simulink model "DiagramaMalhaFechadaForno"  (R2015a)
settings: Solver=ode45  StartTime=0.0  StopTime=15000  RelTol=1e-3
values from neighbouring files (symbols this model uses):
  G = (0.1858/(s + 0.0001438))    [Code50MatLab.m]
libraries: simulink x1
settings Model: Creator=Raian  LastModifiedBy=Emiliano

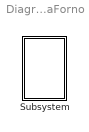
== system DiagramaMalhaFechadaForno ==
  Subsystem : Subsystem

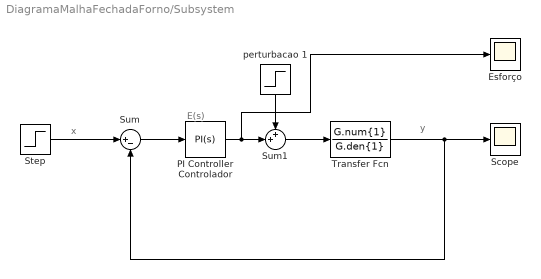
== system DiagramaMalhaFechadaForno/Subsystem ==
  note: E(s)
  note: x
  note: y
  "Esforço " : Scope
  "PI Controller Controlador " : simulink/Continuous/PID Controller  Controller=PI  TimeDomain=Continuous-time  SampleTime=-1  IntegratorMethod=Forward Euler  FilterMethod=Forward Euler  Form=Ideal  UseFilter=on  ControllerParametersSource=internal  P=0.0090  I=0.0001438  D=0  N=100  InitialConditionSource=internal  InitialConditionForIntegrator=0  InitialConditionForFilter=0  ExternalReset=none  LimitOutput=on  UpperSaturationLimit=1  LowerSaturationLimit=0  LinearizeAsGain=on  AntiWindupMode=clamping  Kb=1  TrackingMode=off  Kt=1  PParamMin=[]  PParamMax=[]  IParamMin=[]  IParamMax=[]  DParamMin=[]  DParamMax=[]  NParamMin=[]  NParamMax=[]  KbParamMin=[]  KbParamMax=[]  KtParamMin=[]  KtParamMax=[]  POutMin=[]  POutMax=[]  IOutMin=[]  IOutMax=[]  DOutMin=[]  DOutMax=[]  NOutMin=[]  NOutMax=[]  KbOutMin=[]  KbOutMax=[]  KtOutMin=[]  KtOutMax=[]  IntegratorOutMin=[]  IntegratorOutMax=[]  FilterOutMin=[]  FilterOutMax=[]  SumOutMin=[]  SumOutMax=[]  SumI1OutMin=[]  SumI1OutMax=[]  SumI2OutMin=[]  SumI2OutMax=[]  SumI3OutMin=[]  SumI3OutMax=[]  SumDOutMin=[]  SumDOutMax=[]  SaturationOutMin=[]  SaturationOutMax=[]  IntegratorContinuousStateAttributes=''  IntegratorStateMustResolveToSignalObject=off  IntegratorRTWStateStorageClass=Auto  FilterContinuousStateAttributes=''  FilterStateMustResolveToSignalObject=off  FilterRTWStateStorageClass=Auto  DifferentiatorICPrevScaledInput=0  DifferentiatorOutMin=[]  DifferentiatorOutMax=[]
  "Scope " : Scope
  "Step " : Step  Time=0  After=250
  Sum : Sum  Inputs=|+-
  Sum1 : Sum  Inputs=++|
  "Transfer Fcn " : TransferFcn  Numerator=G.num{1}  Denominator=G.den{1}
  perturbacao 1 : Step  Time=5000  After=-0.1
  wires:
  "Step "/1 -> Sum/1
  Sum/1 -> "PI Controller Controlador "/1
  "Transfer Fcn "/1 -> "Scope "/1, Sum/2
  Sum1/1 -> "Transfer Fcn "/1
  perturbacao 1/1 -> Sum1/1
  "PI Controller Controlador "/1 -> "Esforço "/1, Sum1/2
